simulink model "demand_response"  (Simulink 8.5)
settings: Solver=ode3  StartTime=172800  StopTime=259200  FixedStep=60  RelTol=1e-3
PostLoadFcn:
  | % Force reinitialization of Weather block to create bus definition
  | wBlk = [gcs '/Weather Data'];
  | set_param(wBlk,'initbus',get_param(wBlk,'initbus'));
  | clear('wBlk');
undefined symbols (not defined in the file or in its folder): OHare, USA_IL_Chicago
libraries: simulink x2, mlepLibrary x1, CampusEnergyModeling x1
settings Model: Creator=mwetter  LastModifiedBy=wbernalh  ExtModeAutoUpdateStatusClock=off
settings OptimizationCC: InitFltsAndDblsToZero=on
settings DebuggingCC: SaveWithParameterizedLinksMsg=none  SolverPrmCheckMsg=warning  FcnCallInpInsideContextMsg=UseLocalSettings
settings SFSimCC: SFSimOverflowDetection=off  SFSimEcho=off  SimCtrlC=off  SimIntegrity=off  SimParseCustomCode=off
settings RTWCC: GenerateMakefile=off
settings GRTTargetCC: TargetFcnLib=ansi_tfl_tmw.mat

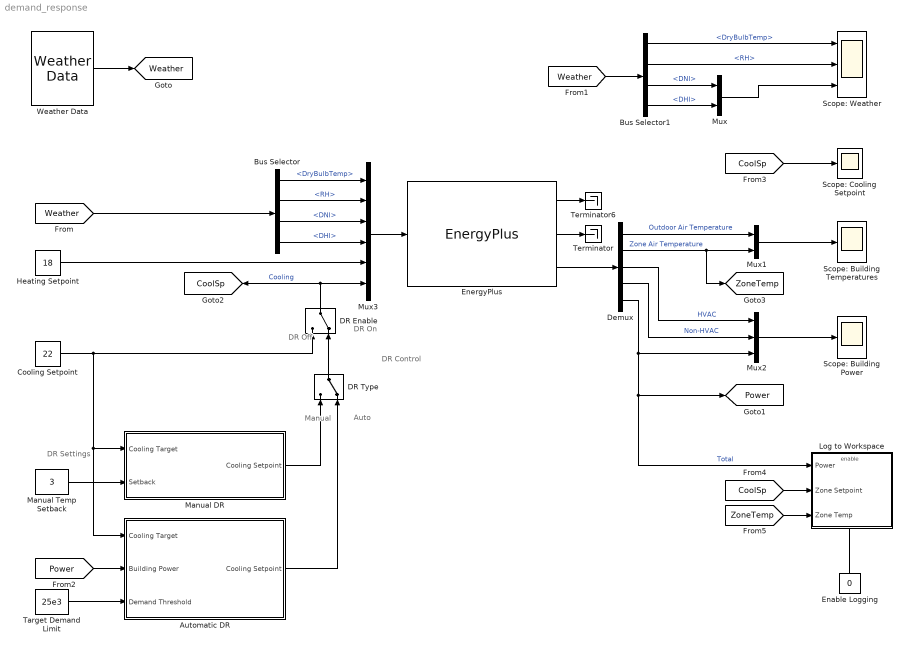
== system demand_response ==
  note: DR Control
  note: Auto
  note: DR Off
  note: DR On
  note: Manual
  note: DR Settings
  Automatic DR : Subsystem
  Bus Selector : BusSelector  OutputSignals=DryBulbTemp,RH,DNI,DHI
  Bus Selector1 : BusSelector  OutputSignals=DryBulbTemp,RH,DNI,DHI
  Cooling Setpoint : Constant  Value=22
  DR Enable : ManualSwitch  CurrentSetting=0
  DR Type : ManualSwitch  CurrentSetting=0
  Demux : Demux  Outputs=5
  Enable Logging : Constant  Value=0
  EnergyPlus : mlepLibrary/EnergyPlus  work_dir=small_office  rel_path=on  fname=small_office.idf  weather_profile=USA_IL_Chicago-OHare.Intl.AP.725300_TMY3  time_step=60  nout=5  timeout=10  mlep_defaults=on  port=0
  Heating Setpoint : Constant  Value=18
  Log to Workspace : Subsystem  TreatAsAtomicUnit=on
  Manual Temp Setback : Constant  Value=3
  Manual DR : Subsystem
  Mux : Mux  Inputs=2
  Mux1 : Mux  Inputs=2
  Mux2 : Mux  Inputs=3
  Mux3 : Mux  Inputs=6
  Scope: Building Power : Scope
      settings: ShowLegends=on  TimeRange=90000  YMin=0  YMax=30000  SaveName=ScopeData2
  Scope: Building Temperatures : Scope
      settings: ShowLegends=on  TimeRange=90000  YMin=5  YMax=35
  Scope: Cooling Setpoint : Scope
      settings: ShowLegends=on  TimeRange=90000  YMin=22  YMax=26  SaveName=ScopeData3
  Scope: Weather : Scope  NumInputPorts=3
      settings: ShowLegends=on  TimeRange=90000  YMin=16~10~0  YMax=34~70~700
  Target Demand Limit : Constant  Value=25e3
  Terminator : Terminator
  Terminator6 : Terminator
  Weather Data : CampusEnergyModeling/Weather/Weather Data  fname=Weather.mat  initbus=on
  tag scope: CoolSp=global, Power=global, Weather=global, ZoneTemp=global
  wires:
  EnergyPlus/3 -> Demux/1
  Weather Data/1 -> [Weather]
  Mux3/1 -> EnergyPlus/1
  [Weather] -> Bus Selector/1
  Bus Selector/1 -> Mux3/1  "<DryBulbTemp>"
  Bus Selector/2 -> Mux3/2  "<RH>"
  Bus Selector/3 -> Mux3/3  "<DNI>"
  Bus Selector/4 -> Mux3/4  "<DHI>"
  Heating Setpoint/1 -> Mux3/5
  EnergyPlus/2 -> Terminator/1
  Bus Selector1/1 -> Scope: Weather/1  "<DryBulbTemp>"
  Bus Selector1/2 -> Scope: Weather/2  "<RH>"
  Bus Selector1/3 -> Mux/1  "<DNI>"
  Bus Selector1/4 -> Mux/2  "<DHI>"
  [Weather] -> Bus Selector1/1
  Mux/1 -> Scope: Weather/3
  EnergyPlus/1 -> Terminator6/1
  Mux1/1 -> Scope: Building Temperatures/1
  Demux/1 -> Mux1/1  "Outdoor Air Temperature"
  Demux/2 -> [ZoneTemp], Mux1/2  "Zone Air Temperature"
  Demux/5 -> Log to Workspace/1(Power), [Power], Mux2/3  "Total"
  Mux2/1 -> Scope: Building Power/1
  Demux/3 -> Mux2/1  "HVAC"
  Demux/4 -> Mux2/2  "Non-HVAC"
  Cooling Setpoint/1 -> DR Enable/1, Manual DR/1(Cooling Target), Automatic DR/1(Cooling Target)
  DR Enable/1 -> [CoolSp], Mux3/6  "Cooling"
  DR Type/1 -> DR Enable/2
  Manual DR/1(Cooling Setpoint) -> DR Type/1
  Automatic DR/1(Cooling Setpoint) -> DR Type/2
  Target Demand Limit/1 -> Automatic DR/3(Demand Threshold)
  [Power] -> Automatic DR/2(Building Power)
  Manual Temp Setback/1 -> Manual DR/2(Setback)
  Enable Logging/1 -> Log to Workspace/Enable
  [CoolSp] -> Scope: Cooling Setpoint/1
  [CoolSp] -> Log to Workspace/2(Zone Setpoint)
  [ZoneTemp] -> Log to Workspace/3(Zone Temp)

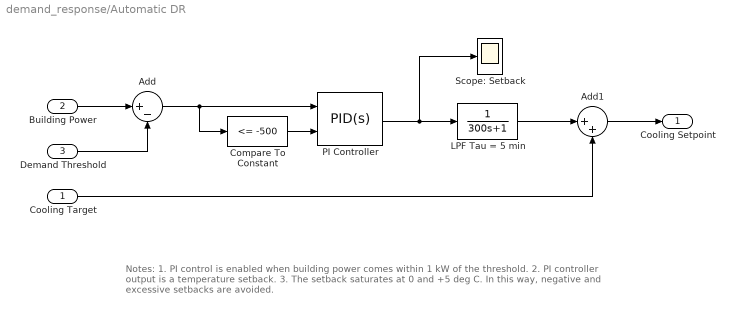
== system demand_response/Automatic DR ==
  note: Notes:
      | 1. PI control is enabled when building power comes within 1 kW of the threshold.
      | 2. PI controller output is a temperature setback.
      | 3. The setback saturates at 0 and +5 deg C. In this way, negative and excessive setbacks are avoided.
  Cooling Target : Inport
  Building Power : Inport  Port=2
  Demand Threshold : Inport  Port=3
  Add : Sum  Inputs=|+-
  Add1 : Sum  Inputs=|++
  Compare To Constant : simulink/Logic and Bit Operations/Compare To Constant  relop=<=  const=-500  OutDataTypeStr=boolean
  LPF Tau = 5 min : TransferFcn  Denominator=[300 1]
  PI Controller : simulink/Continuous/PID Controller  Controller=PID  TimeDomain=Continuous-time  SampleTime=-1  IntegratorMethod=Forward Euler  FilterMethod=Forward Euler  Form=Parallel  UseFilter=on  ControllerParametersSource=internal  P=2e-4  I=2e-6  D=0  N=100  InitialConditionSource=internal  InitialConditionForIntegrator=0  InitialConditionForFilter=0  ExternalReset=level  LimitOutput=on  UpperSaturationLimit=3  LowerSaturationLimit=0  LinearizeAsGain=on  AntiWindupMode=none  Kb=1  TrackingMode=off  Kt=1  PParamMin=[]  PParamMax=[]  IParamMin=[]  IParamMax=[]  DParamMin=[]  DParamMax=[]  NParamMin=[]  NParamMax=[]  KbParamMin=[]  KbParamMax=[]  KtParamMin=[]  KtParamMax=[]  POutMin=[]  POutMax=[]  IOutMin=[]  IOutMax=[]  DOutMin=[]  DOutMax=[]  NOutMin=[]  NOutMax=[]  KbOutMin=[]  KbOutMax=[]  KtOutMin=[]  KtOutMax=[]  IntegratorOutMin=[]  IntegratorOutMax=[]  FilterOutMin=[]  FilterOutMax=[]  SumOutMin=[]  SumOutMax=[]  SumI1OutMin=[]  SumI1OutMax=[]  SumI2OutMin=[]  SumI2OutMax=[]  SumI3OutMin=[]  SumI3OutMax=[]  SumDOutMin=[]  SumDOutMax=[]  SaturationOutMin=[]  SaturationOutMax=[]  IntegratorContinuousStateAttributes=''  IntegratorStateMustResolveToSignalObject=off  IntegratorRTWStateStorageClass=Auto  FilterContinuousStateAttributes=''  FilterStateMustResolveToSignalObject=off  FilterRTWStateStorageClass=Auto  DifferentiatorICPrevScaledInput=0  DifferentiatorOutMin=[]  DifferentiatorOutMax=[]
  Scope: Setback : Scope
      settings: ShowLegends=on  TimeRange=90000  YMin=0  YMax=4  SaveName=ScopeData4
  Cooling Setpoint : Outport
  wires:
  Building Power/1 -> Add/1
  Demand Threshold/1 -> Add/2
  Cooling Target/1 -> Add1/2
  Add/1 -> Compare To Constant/1, PI Controller/1
  Add1/1 -> Cooling Setpoint/1
  LPF Tau = 5 min/1 -> Add1/1
  PI Controller/1 -> Scope: Setback/1, LPF Tau = 5 min/1
  Compare To Constant/1 -> PI Controller/2

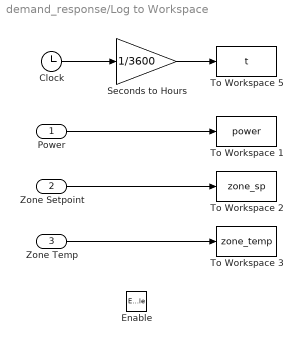
== system demand_response/Log to Workspace ==
  Power : Inport
  Zone Setpoint : Inport  Port=2
  Zone Temp : Inport  Port=3
  Enable : EnablePort
  Clock : Clock
  Seconds to Hours : Gain  Gain=1/3600
  To Workspace 1 : ToWorkspace  VariableName=power  SampleTime=-1
  To Workspace 2 : ToWorkspace  VariableName=zone_sp  SampleTime=-1
  To Workspace 3 : ToWorkspace  VariableName=zone_temp  SampleTime=-1
  To Workspace 5 : ToWorkspace  VariableName=t  SampleTime=-1
  wires:
  Power/1 -> To Workspace 1/1
  Zone Setpoint/1 -> To Workspace 2/1
  Zone Temp/1 -> To Workspace 3/1
  Clock/1 -> Seconds to Hours/1
  Seconds to Hours/1 -> To Workspace 5/1

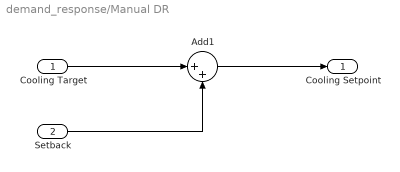
== system demand_response/Manual DR ==
  Cooling Target : Inport
  Setback : Inport  Port=2
  Add1 : Sum  Inputs=|++
  Cooling Setpoint : Outport
  wires:
  Cooling Target/1 -> Add1/1
  Setback/1 -> Add1/2
  Add1/1 -> Cooling Setpoint/1
